simulink model "soc_WLAN_fpga"  (R2024b)
settings: Solver=FixedStepDiscrete  StartTime=0.0  StopTime=stopTime  RelTol=1e-3
PreLoadFcn:
  | addpath(fullfile(matlabroot,'toolbox','whdl','whdlexamples','whdlexamples'));
InitFcn:
  | addpath(fullfile(matlabroot,'toolbox','whdl','whdlexamples','whdlexamples'));
model workspace (MAT data in the model file):
  socvcb : containers.Map (value not decoded)
undefined symbols (not defined in the file): Add, bitRatePerOfdmSym, chanBW, coe, cpLen, dataUpsampleFactor, DelayValMaxNsdMinusLastPilotSc, DescramblerInitialSeed, designMultirateFIR, fftLen, filterLatency, filterUpsampleFactor, Fs, Hd, HT_MFMCS0, HT_MFMCS1, HT_MFMCS2, HT_MFMCS3, HT_MFMCS4, HT_MFMCS5, HT_MFMCS6, HT_MFMCS7, HTUnUsedScInd, inputSamplingRate, interp_coeff, maxPilotRefCounterVale, maxPilotsRef, maxPilotsRefNonHT, Ncol_HT, Ncol_NonHT, noDataSubCarriers, Non_HTMCS0, Non_HTMCS1, Non_HTMCS2, Non_HTMCS3, Non_HTMCS4, Non_HTMCS5, Non_HTMCS6, Non_HTMCS7, Nrow_HT, Nrow_NonHT, numDSC_HT, numDSC_HT_vhtSigB, numDSC_NonHT, numDscHT, numDscNonHT, numOfBitsPerOFDMSym, numOfDataBitsPerOFDMSym, numPilots, numScHT, numSCS_HT, numSCS_NonHT, pnSeq, QAM, rxDownsampleFactor, secondPIdx_HT, secondPIdx_NonHT, Shift, VHTMCS0, VHTMCS1 ... (+7)
libraries: hdlsllib x267, simulink x210, dspsigops x22, whdlutilities x10, whdlmod x9, dsphdlfiltering2 x5, dsphdlmathfun2 x4, whdledac x3, hwlogicconnlib x2, commhdlcrc x2, dsphdlsigops2 x2
(part 7 of 14)

== system soc_WLAN_fpga/WLAN/WLAN HDL/WLAN_Tx_Rx/WLAN_Rx/WLANHDLReceiver/DataRecovery/Decoder/Depuncturer/DepuncturerCtrlGen ==
  format : Inport
  vitInputLen : Inport  Port=2
  rstIn : Inport  Port=3
  validIn : Inport  Port=4
  Add : Sum  Inputs=+-
  Compare To Constant : simulink/Logic and Bit Operations/Compare To Constant  relop===  const=2  OutDataTypeStr=boolean
  Compare To Constant1 : simulink/Logic and Bit Operations/Compare To Constant  relop===  const=numDSC_HT_vhtSigB-1  OutDataTypeStr=boolean
  Compare To Constant2 : simulink/Logic and Bit Operations/Compare To Constant  relop===  const=numDSC_HT_vhtSigB  OutDataTypeStr=boolean
  Compare To Constant4 : simulink/Logic and Bit Operations/Compare To Constant  relop=<=  const=numDSC_HT_vhtSigB-1  OutDataTypeStr=boolean
  Compare To Zero : simulink/Logic and Bit Operations/Compare To Zero  relop===  OutDataTypeStr=boolean
  Constant : Constant  Value=fi(1,0,1,0)  SampleTime=-1
  Constant1 : Constant  Value=numDSC_HT_vhtSigB  OutDataTypeStr=fixdt(0,17,0)  SampleTime=-1
  HDL Counter : hdlsllib/Sources/HDL Counter  CountType=Count limited  CountInit=0  CountStep=1  CountMax=65535  CountFromType=Initial value  CountFrom=0  CountResetPort=on  CountLoadPort=off  CountEnbPort=on  CountDirPort=off  CountHitOutputPort=off  CountDataType=Unsigned  CountWordLen=16  CountFracLen=0  CountSampTime=1
  Logical Operator{,1..2,5,7} (5 alike) : Logic  AllPortsSameDT=off  OutDataTypeStr=boolean
  Logical Operator3 : Logic  Operator=OR  AllPortsSameDT=off  OutDataTypeStr=boolean
  Logical Operator6 : Logic  Operator=OR  AllPortsSameDT=off  OutDataTypeStr=boolean
  Relational Operator : RelationalOperator  Operator===  OutDataTypeStr=boolean  RndMeth=Simplest  InputSameDT=off
  Switch2 : Switch  Criteria=u2 > Threshold  SaturateOnIntegerOverflow=off  InputSameDT=off
  start : Outport
  end : Outport  Port=2
  wires:
  Switch2/1 -> Add/1
  Logical Operator/1 -> end/1
  Logical Operator1/1 -> start/1
  vitInputLen/1 -> Switch2/3
  validIn/1 -> Logical Operator1/2, Logical Operator/2, HDL Counter/2
  rstIn/1 -> HDL Counter/1
  Logical Operator2/1 -> Logical Operator3/1
  Constant/1 -> Add/2
  HDL Counter/1 -> Compare To Zero/1, Compare To Constant4/1, Relational Operator/2, Compare To Constant2/1, Compare To Constant1/1
  Constant1/1 -> Switch2/1
  Logical Operator6/1 -> Logical Operator1/1
  Compare To Constant2/1 -> Logical Operator5/2
  Logical Operator5/1 -> Logical Operator6/1
  Relational Operator/1 -> Logical Operator3/2
  Compare To Zero/1 -> Logical Operator6/2
  Compare To Constant4/1 -> Logical Operator7/1
  format/1 -> Compare To Constant/1
  Logical Operator3/1 -> Logical Operator/1
  Logical Operator7/1 -> Switch2/2
  Compare To Constant1/1 -> Logical Operator2/2
  Add/1 -> Relational Operator/1
  Compare To Constant/1 -> Logical Operator7/2, Logical Operator5/1, Logical Operator2/1

== system soc_WLAN_fpga/WLAN/WLAN HDL/WLAN_Tx_Rx/WLAN_Rx/WLANHDLReceiver/DataRecovery/Decoder/vhtSigB/vhtSigBDecoding ==
  note: Calculating PSDU len for VHT frame using initial 25bits of VHT SigB
  note: Dectecting CRC on first 19 bits
  MCS : Inport
  rst : Inport  Port=2
  bit : Inport  Port=3
  format : Inport  Port=4
  valid : Inport  Port=5
  Compare To Constant : simulink/Logic and Bit Operations/Compare To Constant  relop===  const=2  OutDataTypeStr=boolean
  Compare To Constant1 : simulink/Logic and Bit Operations/Compare To Constant  relop=<=  const=25  OutDataTypeStr=boolean
  Compare To Constant2 : simulink/Logic and Bit Operations/Compare To Constant  relop=<=  const=19+double(chanBW==2)  OutDataTypeStr=boolean
  Compare To Constant3 : simulink/Logic and Bit Operations/Compare To Constant  relop===  const=0  OutDataTypeStr=boolean
  Compare To Constant4 : simulink/Logic and Bit Operations/Compare To Constant  relop===  const=19+double(chanBW==2)  OutDataTypeStr=boolean
  Compare To Constant5 : simulink/Logic and Bit Operations/Compare To Constant  relop=>  const=19+double(chanBW==2)  OutDataTypeStr=boolean
  Delay : Delay  DelayLength=1
  Delay1 : Delay  DelayLength=1
  Delay3 : Delay  DelayLength=1
  Delay5 : Delay  DelayLength=9
  General CRC Generator HDL Optimized : commhdlcrc/General CRC Generator HDL Optimized  Polynomial=[1 0 0 0 0 0 1 1 1]  InitialState=1  DirectMethod=on  ReflectInput=off  ReflectCRCChecksum=off  FinalXORValue=1  SimulateUsing=Code generation
  HDL Counter : hdlsllib/Sources/HDL Counter  CountType=Count limited  CountInit=0  CountStep=1  CountMax=65535  CountFromType=Initial value  CountFrom=0  CountResetPort=on  CountLoadPort=off  CountEnbPort=on  CountDirPort=off  CountHitOutputPort=off  CountDataType=Unsigned  CountWordLen=16  CountFracLen=0  CountSampTime=1
  HDL Counter1 : hdlsllib/Sources/HDL Counter  CountType=Count limited  CountInit=0  CountStep=1  CountMax=65535  CountFromType=Initial value  CountFrom=0  CountResetPort=on  CountLoadPort=off  CountEnbPort=on  CountDirPort=off  CountHitOutputPort=off  CountDataType=Unsigned  CountWordLen=16  CountFracLen=0  CountSampTime=1
  Logical Operator{,1..3} (4 alike) : Logic  Inputs=3  AllPortsSameDT=off  OutDataTypeStr=boolean
  Logical Operator4 : Logic  AllPortsSameDT=off  OutDataTypeStr=boolean
  Shift Arithmetic : ArithShift  BitShiftNumber=2  BitShiftDirection=Left
  Terminator1 : Terminator
  Terminator3 : Terminator
  To Workspace : ToWorkspace  VariableName=vhtSigBits  SampleTime=-1
      settings: Save2DSignal=2-D array (concatenate along first dimension)
  To Workspace1 : ToWorkspace  VariableName=vhtSigBitsV  SampleTime=-1
      settings: Save2DSignal=2-D array (concatenate along first dimension)
  interpretVHTSigB : MATLAB Function  TreatAsAtomicUnit=on
  vitInputLenCalc : Subsystem
  vitInputLen : Outport
  psduLen : Outport  Port=2
  vhtCRCRefBits : Outport  Port=3
  vhtCRCRefBitValid : Outport  Port=4
  vhtSigBBitVld : Outport  Port=5
  wires:
  format/1 -> Compare To Constant/1
  valid/1 -> Logical Operator3/2, Logical Operator1/2, Logical Operator2/2, Logical Operator/3, HDL Counter/2
  rst/1 -> HDL Counter1/1, interpretVHTSigB/4(reset), HDL Counter/1
  bit/1 -> General CRC Generator HDL Optimized/1, To Workspace/1, interpretVHTSigB/1(bit)
  interpretVHTSigB/1(psduLen) -> Shift Arithmetic/1
  Compare To Constant1/1 -> Logical Operator/2
  HDL Counter/1 -> Compare To Constant1/1, Compare To Constant2/1, Compare To Constant3/1, Compare To Constant4/1, interpretVHTSigB/3(countVal)
  Compare To Constant2/1 -> Logical Operator1/3
  Logical Operator1/1 -> General CRC Generator HDL Optimized/4
  Compare To Constant3/1 -> Logical Operator2/3
  Logical Operator2/1 -> General CRC Generator HDL Optimized/2
  Logical Operator3/1 -> General CRC Generator HDL Optimized/3
  Compare To Constant4/1 -> Logical Operator3/3
  Compare To Constant/1 -> Logical Operator2/1, Logical Operator1/1, Logical Operator3/1, Logical Operator/1
  General CRC Generator HDL Optimized/4 -> Logical Operator4/1, HDL Counter1/2
  vitInputLenCalc/2(decoderInpLen) -> vitInputLen/1
  vitInputLenCalc/1(updatedPsduLen) -> psduLen/1
  MCS/1 -> Delay/1
  Shift Arithmetic/1 -> Delay1/1
  Logical Operator/1 -> Delay3/1, To Workspace1/1, interpretVHTSigB/2(validIn)
  Delay/1 -> vitInputLenCalc/1(MCS)
  Delay1/1 -> vitInputLenCalc/2(psduLen)
  Delay3/1 -> Delay5/1
  Delay5/1 -> vhtSigBBitVld/1
  General CRC Generator HDL Optimized/2 -> Terminator1/1
  General CRC Generator HDL Optimized/3 -> Terminator3/1
  General CRC Generator HDL Optimized/1 -> vhtCRCRefBits/1
  HDL Counter1/1 -> Compare To Constant5/1
  Compare To Constant5/1 -> Logical Operator4/2
  Logical Operator4/1 -> vhtCRCRefBitValid/1

== system soc_WLAN_fpga/WLAN/WLAN HDL/WLAN_Tx_Rx/WLAN_Rx/WLANHDLReceiver/DataRecovery/Deinterleaver/DeInterleaver_HT/Stage 2 16QAM  ==
  note: Give null output if valid is LOW
  dataIn : Inport
  startIn : Inport  Port=2
  endIn : Inport  Port=3
  validIn : Inport  Port=4
  Constant : Constant  Value=0  OutDataTypeStr=Inherit: Inherit via back propagation  SampleTime=-1
  Delay{1,3..6,9..11} (8 alike) : Delay  DelayLength=1
  Delay12 : Delay  DelayLength=7
  Delay13 : Delay  DelayLength=7
  Delay14 : Delay  DelayLength=7
  Delay{2,15..17} (4 alike) : Delay
  Delay7 : Delay  DelayLength=1  InitialCondition=true
  Delay8 : Delay  DelayLength=1  InitialCondition=true
  Generate Ready : Subsystem
  Logical Operator : Logic  IconShape=distinctive  AllPortsSameDT=off  OutDataTypeStr=boolean
  RAM : hdlsllib/HDL RAMs/Simple Dual Port RAM  ram_size=nextpow2(2*maxBlkSize)
  Read Logic : Subsystem
  Store Block Lengths : hdlsllib/HDL RAMs/HDL FIFO  fifo_size=4  mode=Classic  ratio=1  push_msg=Warning  pop_msg=Ignore  show_empty=off  show_full=off  show_num=on  LabelModeActiveChoice_Mode=Classic  rst_port=off
  Switch : Switch  Criteria=u2 ~= 0  SaturateOnIntegerOverflow=off
  Write Logic : Subsystem
  dataOut : Outport
  startOut : Outport  Port=2
  endOut : Outport  Port=3
  validOut : Outport  Port=4
  ready : Outport  Port=5
  wires:
  Delay17/1 -> Delay14/1
  Delay16/1 -> Delay12/1
  Delay15/1 -> Delay13/1
  Delay14/1 -> RAM/1
  Delay12/1 -> RAM/2
  Delay13/1 -> RAM/3
  Constant/1 -> Switch/3
  Switch/1 -> dataOut/1
  RAM/1 -> Switch/1
  Generate Ready/1(ready) -> ready/1, [ready]
  Read Logic/6(advPop) -> Generate Ready/1(advPop)
  Write Logic/5(endReady) -> Generate Ready/4(endReady)
  Delay7/1 -> Logical Operator/2
  validIn/1 -> Logical Operator/1
  Logical Operator/1 -> Write Logic/2(valid)
  [ready] -> Delay7/1
  Read Logic/5(pop) -> [b]
  Delay6/1 -> startOut/1
  Delay10/1 -> validOut/1, Switch/2
  Delay5/1 -> endOut/1
  Delay11/1 -> Store Block Lengths/2
  Delay9/1 -> Store Block Lengths/1
  Delay4/1 -> Delay15/1
  Delay3/1 -> Delay16/1
  Delay1/1 -> Delay17/1
  Delay8/1 -> Store Block Lengths/3, Generate Ready/3(pop)
  [b] -> Delay8/1
  Read Logic/3(end) -> Delay5/1
  Read Logic/2(start) -> Delay6/1
  Read Logic/1(rdAddr) -> RAM/4
  Store Block Lengths/1 -> Read Logic/1(fifoData)
  Read Logic/4(valid) -> Delay10/1
  Write Logic/4(endOut) -> Delay11/1
  Write Logic/3(count) -> Delay9/1
  Write Logic/2(wrValid) -> Delay4/1
  Write Logic/1(wrAddr) -> Delay3/1
  endIn/1 -> Write Logic/3(end)
  startIn/1 -> Write Logic/1(start)
  Delay2/1 -> Delay1/1
  dataIn/1 -> Delay2/1
  Store Block Lengths/2 -> Read Logic/2(fifoCount), Generate Ready/2(fifoCount)

== system soc_WLAN_fpga/WLAN/WLAN HDL/WLAN_Tx_Rx/WLAN_Rx/WLANHDLReceiver/DataRecovery/Deinterleaver/DeInterleaver_HT/Stage 2 64QAM ==
  note: Give null output if valid is LOW
  dataIn : Inport
  startIn : Inport  Port=2
  endIn : Inport  Port=3
  validIn : Inport  Port=4
  Constant : Constant  Value=0  OutDataTypeStr=Inherit: Inherit via back propagation  SampleTime=-1
  Delay{1,3..6,9..11} (8 alike) : Delay  DelayLength=1
  Delay12 : Delay  DelayLength=7
  Delay13 : Delay  DelayLength=7
  Delay14 : Delay  DelayLength=7
  Delay{2,15..17} (4 alike) : Delay
  Delay7 : Delay  DelayLength=1  InitialCondition=true
  Delay8 : Delay  DelayLength=1  InitialCondition=true
  Generate Ready : Subsystem
  Logical Operator : Logic  IconShape=distinctive  AllPortsSameDT=off  OutDataTypeStr=boolean
  RAM : hdlsllib/HDL RAMs/Simple Dual Port RAM  ram_size=nextpow2(2*maxBlkSize)
  Read Logic : Subsystem
  Store Block Lengths : hdlsllib/HDL RAMs/HDL FIFO  fifo_size=4  mode=Classic  ratio=1  push_msg=Warning  pop_msg=Ignore  show_empty=off  show_full=off  show_num=on  LabelModeActiveChoice_Mode=Classic  rst_port=off
  Switch : Switch  Criteria=u2 ~= 0  SaturateOnIntegerOverflow=off
  Write Logic : Subsystem
  dataOut : Outport
  startOut : Outport  Port=2
  endOut : Outport  Port=3
  validOut : Outport  Port=4
  ready : Outport  Port=5
  wires:
  Delay17/1 -> Delay14/1
  Delay16/1 -> Delay12/1
  Delay15/1 -> Delay13/1
  Delay14/1 -> RAM/1
  Delay12/1 -> RAM/2
  Delay13/1 -> RAM/3
  Constant/1 -> Switch/3
  Switch/1 -> dataOut/1
  RAM/1 -> Switch/1
  Generate Ready/1(ready) -> ready/1, [ready]
  Read Logic/6(advPop) -> Generate Ready/1(advPop)
  Write Logic/5(endReady) -> Generate Ready/4(endReady)
  Delay7/1 -> Logical Operator/2
  validIn/1 -> Logical Operator/1
  Logical Operator/1 -> Write Logic/2(valid)
  [ready] -> Delay7/1
  Read Logic/5(pop) -> [b]
  Delay6/1 -> startOut/1
  Delay10/1 -> validOut/1, Switch/2
  Delay5/1 -> endOut/1
  Delay11/1 -> Store Block Lengths/2
  Delay9/1 -> Store Block Lengths/1
  Delay4/1 -> Delay15/1
  Delay3/1 -> Delay16/1
  Delay1/1 -> Delay17/1
  Delay8/1 -> Store Block Lengths/3, Generate Ready/3(pop)
  [b] -> Delay8/1
  Read Logic/3(end) -> Delay5/1
  Read Logic/2(start) -> Delay6/1
  Read Logic/1(rdAddr) -> RAM/4
  Store Block Lengths/1 -> Read Logic/1(fifoData)
  Read Logic/4(valid) -> Delay10/1
  Write Logic/4(endOut) -> Delay11/1
  Write Logic/3(count) -> Delay9/1
  Write Logic/2(wrValid) -> Delay4/1
  Write Logic/1(wrAddr) -> Delay3/1
  endIn/1 -> Write Logic/3(end)
  startIn/1 -> Write Logic/1(start)
  Delay2/1 -> Delay1/1
  dataIn/1 -> Delay2/1
  Store Block Lengths/2 -> Read Logic/2(fifoCount), Generate Ready/2(fifoCount)

== system soc_WLAN_fpga/WLAN/WLAN HDL/WLAN_Tx_Rx/WLAN_Rx/WLANHDLReceiver/DataRecovery/Deinterleaver/DeInterleaver_HT/Stage 2 BPSK ==
  note: Give null output if valid is LOW
  dataIn : Inport
  startIn : Inport  Port=2
  endIn : Inport  Port=3
  validIn : Inport  Port=4
  Constant : Constant  Value=0  OutDataTypeStr=Inherit: Inherit via back propagation  SampleTime=-1
  Delay{1,3..6,9..11} (8 alike) : Delay  DelayLength=1
  Delay12 : Delay  DelayLength=7
  Delay13 : Delay  DelayLength=7
  Delay14 : Delay  DelayLength=7
  Delay{2,15..17} (4 alike) : Delay
  Delay7 : Delay  DelayLength=1  InitialCondition=true
  Delay8 : Delay  DelayLength=1  InitialCondition=true
  Generate Ready : Subsystem
  Logical Operator : Logic  IconShape=distinctive  AllPortsSameDT=off  OutDataTypeStr=boolean
  RAM : hdlsllib/HDL RAMs/Simple Dual Port RAM  ram_size=nextpow2(2*maxBlkSize)
  Read Logic : Subsystem
  Store Block Lengths : hdlsllib/HDL RAMs/HDL FIFO  fifo_size=4  mode=Classic  ratio=1  push_msg=Warning  pop_msg=Ignore  show_empty=off  show_full=off  show_num=on  LabelModeActiveChoice_Mode=Classic  rst_port=off
  Switch : Switch  Criteria=u2 ~= 0  SaturateOnIntegerOverflow=off
  Write Logic : Subsystem
  dataOut : Outport
  startOut : Outport  Port=2
  endOut : Outport  Port=3
  validOut : Outport  Port=4
  ready : Outport  Port=5
  wires:
  Delay17/1 -> Delay14/1
  Delay16/1 -> Delay12/1
  Delay15/1 -> Delay13/1
  Delay14/1 -> RAM/1
  Delay12/1 -> RAM/2
  Delay13/1 -> RAM/3
  Constant/1 -> Switch/3
  Switch/1 -> dataOut/1
  RAM/1 -> Switch/1
  Generate Ready/1(ready) -> ready/1, [ready]
  Read Logic/6(advPop) -> Generate Ready/1(advPop)
  Write Logic/5(endReady) -> Generate Ready/4(endReady)
  Delay7/1 -> Logical Operator/2
  validIn/1 -> Logical Operator/1
  Logical Operator/1 -> Write Logic/2(valid)
  [ready] -> Delay7/1
  Read Logic/5(pop) -> [b]
  Delay6/1 -> startOut/1
  Delay10/1 -> validOut/1, Switch/2
  Delay5/1 -> endOut/1
  Delay11/1 -> Store Block Lengths/2
  Delay9/1 -> Store Block Lengths/1
  Delay4/1 -> Delay15/1
  Delay3/1 -> Delay16/1
  Delay1/1 -> Delay17/1
  Delay8/1 -> Store Block Lengths/3, Generate Ready/3(pop)
  [b] -> Delay8/1
  Read Logic/3(end) -> Delay5/1
  Read Logic/2(start) -> Delay6/1
  Read Logic/1(rdAddr) -> RAM/4
  Store Block Lengths/1 -> Read Logic/1(fifoData)
  Read Logic/4(valid) -> Delay10/1
  Write Logic/4(endOut) -> Delay11/1
  Write Logic/3(count) -> Delay9/1
  Write Logic/2(wrValid) -> Delay4/1
  Write Logic/1(wrAddr) -> Delay3/1
  endIn/1 -> Write Logic/3(end)
  startIn/1 -> Write Logic/1(start)
  Delay2/1 -> Delay1/1
  dataIn/1 -> Delay2/1
  Store Block Lengths/2 -> Read Logic/2(fifoCount), Generate Ready/2(fifoCount)

== system soc_WLAN_fpga/WLAN/WLAN HDL/WLAN_Tx_Rx/WLAN_Rx/WLANHDLReceiver/DataRecovery/Deinterleaver/DeInterleaver_HT/Stage 2 QPSK ==
  note: Give null output if valid is LOW
  dataIn : Inport
  startIn : Inport  Port=2
  endIn : Inport  Port=3
  validIn : Inport  Port=4
  Constant : Constant  Value=0  OutDataTypeStr=Inherit: Inherit via back propagation  SampleTime=-1
  Delay{1,3..6,9..11} (8 alike) : Delay  DelayLength=1
  Delay12 : Delay  DelayLength=7
  Delay13 : Delay  DelayLength=7
  Delay14 : Delay  DelayLength=7
  Delay{2,15..17} (4 alike) : Delay
  Delay7 : Delay  DelayLength=1  InitialCondition=true
  Delay8 : Delay  DelayLength=1  InitialCondition=true
  Generate Ready : Subsystem
  Logical Operator : Logic  IconShape=distinctive  AllPortsSameDT=off  OutDataTypeStr=boolean
  RAM : hdlsllib/HDL RAMs/Simple Dual Port RAM  ram_size=nextpow2(2*maxBlkSize)
  Read Logic : Subsystem
  Store Block Lengths : hdlsllib/HDL RAMs/HDL FIFO  fifo_size=4  mode=Classic  ratio=1  push_msg=Warning  pop_msg=Ignore  show_empty=off  show_full=off  show_num=on  LabelModeActiveChoice_Mode=Classic  rst_port=off
  Switch : Switch  Criteria=u2 ~= 0  SaturateOnIntegerOverflow=off
  Write Logic : Subsystem
  dataOut : Outport
  startOut : Outport  Port=2
  endOut : Outport  Port=3
  validOut : Outport  Port=4
  ready : Outport  Port=5
  wires:
  Delay17/1 -> Delay14/1
  Delay16/1 -> Delay12/1
  Delay15/1 -> Delay13/1
  Delay14/1 -> RAM/1
  Delay12/1 -> RAM/2
  Delay13/1 -> RAM/3
  Constant/1 -> Switch/3
  Switch/1 -> dataOut/1
  RAM/1 -> Switch/1
  Generate Ready/1(ready) -> ready/1, [ready]
  Read Logic/6(advPop) -> Generate Ready/1(advPop)
  Write Logic/5(endReady) -> Generate Ready/4(endReady)
  Delay7/1 -> Logical Operator/2
  validIn/1 -> Logical Operator/1
  Logical Operator/1 -> Write Logic/2(valid)
  [ready] -> Delay7/1
  Read Logic/5(pop) -> [b]
  Delay6/1 -> startOut/1
  Delay10/1 -> validOut/1, Switch/2
  Delay5/1 -> endOut/1
  Delay11/1 -> Store Block Lengths/2
  Delay9/1 -> Store Block Lengths/1
  Delay4/1 -> Delay15/1
  Delay3/1 -> Delay16/1
  Delay1/1 -> Delay17/1
  Delay8/1 -> Store Block Lengths/3, Generate Ready/3(pop)
  [b] -> Delay8/1
  Read Logic/3(end) -> Delay5/1
  Read Logic/2(start) -> Delay6/1
  Read Logic/1(rdAddr) -> RAM/4
  Store Block Lengths/1 -> Read Logic/1(fifoData)
  Read Logic/4(valid) -> Delay10/1
  Write Logic/4(endOut) -> Delay11/1
  Write Logic/3(count) -> Delay9/1
  Write Logic/2(wrValid) -> Delay4/1
  Write Logic/1(wrAddr) -> Delay3/1
  endIn/1 -> Write Logic/3(end)
  startIn/1 -> Write Logic/1(start)
  Delay2/1 -> Delay1/1
  dataIn/1 -> Delay2/1
  Store Block Lengths/2 -> Read Logic/2(fifoCount), Generate Ready/2(fifoCount)

== system soc_WLAN_fpga/WLAN/WLAN HDL/WLAN_Tx_Rx/WLAN_Rx/WLANHDLReceiver/DataRecovery/Deinterleaver/DeInterleaver_HT/Stage1 ==
  wr_din : Inport
  enb : Inport  Port=2
  bps : Inport  Port=3
  rst : Inport  Port=4
  numSCs : Inport  Port=5
  2-D Lookup Table : Lookup_n-D  BreakpointsForDimension1=1:4  BreakpointsForDimension2=0:length(secondPIdx_HT)-1  IndexSearchMethod=Evenly spaced points  Table=uint16(secondPIdx_HT-1)  ExtrapMethod=Clip  UseLastTableValue=on  InternalRulePriority=Speed  OutDataTypeStr=uint16  RndMeth=Simplest
      settings: InputPortMap=u0,u1
  Compare To Constant1 : simulink/Logic and Bit Operations/Compare To Constant  relop===  const=0  OutDataTypeStr=boolean
  Compare To Zero : simulink/Logic and Bit Operations/Compare To Zero  relop=>  OutDataTypeStr=boolean
  Constant : Constant  OutDataTypeStr=uint16  SampleTime=-1
  Delay : Delay  DelayLength=52
  Delay1 : Delay  DelayLength=1  InputProcessing=Columns as channels (frame based)
  Delay{2..9} (8 alike) : Delay  DelayLength=1
  HDL Counter : hdlsllib/Sources/HDL Counter  CountType=Count limited  CountInit=0  CountStep=1  CountMax=length(secondPIdx_HT)-1  CountFromType=Initial value  CountFrom=0  CountResetPort=on  CountLoadPort=off  CountEnbPort=on  CountDirPort=off  CountHitOutputPort=off  CountDataType=Unsigned  CountWordLen=16  CountFracLen=0  CountSampTime=1
  HDL Counter1 : hdlsllib/Sources/HDL Counter  CountType=Count limited  CountInit=0  CountStep=1  CountMax=1  CountFromType=Initial value  CountFrom=0  CountResetPort=on  CountLoadPort=off  CountEnbPort=on  CountDirPort=off  CountHitOutputPort=off  CountDataType=Unsigned  CountWordLen=1  CountFracLen=0  CountSampTime=1
  HDL Counter2 : hdlsllib/Sources/HDL Counter  CountType=Count limited  CountInit=0  CountStep=1  CountMax=length(secondPIdx_HT)-1  CountFromType=Initial value  CountFrom=0  CountResetPort=on  CountLoadPort=on  CountEnbPort=on  CountDirPort=off  CountHitOutputPort=off  CountDataType=Unsigned  CountWordLen=16  CountFracLen=0  CountSampTime=1
  Logical Operator : Logic  AllPortsSameDT=off  OutDataTypeStr=boolean
  Logical Operator1 : Logic  AllPortsSameDT=off  OutDataTypeStr=boolean
  Logical Operator2 : Logic  Operator=NOT  AllPortsSameDT=off  OutDataTypeStr=boolean
  Logical Operator3 : Logic  Operator=OR  AllPortsSameDT=off  OutDataTypeStr=boolean
  Logical Operator4 : Logic  Operator=OR  AllPortsSameDT=off  OutDataTypeStr=boolean
  Logical Operator5 : Logic  Operator=OR  AllPortsSameDT=off  OutDataTypeStr=boolean
  Logical Operator6 : Logic  AllPortsSameDT=off  OutDataTypeStr=boolean
  Relational Operator : RelationalOperator  Operator===  OutDataTypeStr=boolean  RndMeth=Simplest  InputSameDT=off
  Relational Operator1 : RelationalOperator  Operator===  OutDataTypeStr=boolean  RndMeth=Simplest  InputSameDT=off
  Simple Dual Port RAM : hdlsllib/HDL RAMs/Simple Dual Port RAM  ram_size=16
  Simple Dual Port RAM1 : hdlsllib/HDL RAMs/Simple Dual Port RAM  ram_size=16
  Switch : Switch  Criteria=u2 > Threshold  SaturateOnIntegerOverflow=off  InputSameDT=off
  dataOut : Outport
  validOut : Outport  Port=2
  wires:
  enb/1 -> HDL Counter/2, Logical Operator6/1, Logical Operator/1, Logical Operator1/1
  Simple Dual Port RAM/1 -> Switch/1
  bps/1 -> 2-D Lookup Table/1
  HDL Counter/1 -> Delay3/1, Relational Operator/1, Delay6/1
  HDL Counter1/1 -> Compare To Constant1/1
  wr_din/1 -> Delay2/1
  Relational Operator/1 -> Logical Operator6/2
  Logical Operator1/1 -> Delay7/1
  2-D Lookup Table/1 -> Delay8/1
  rst/1 -> HDL Counter1/1, Logical Operator4/1, Logical Operator3/1
  Simple Dual Port RAM1/1 -> Switch/3
  Logical Operator/1 -> Delay4/1
  Switch/1 -> dataOut/1
  Delay1/1 -> validOut/1
  HDL Counter2/1 -> Compare To Zero/1, Relational Operator1/1, 2-D Lookup Table/2
  Compare To Constant1/1 -> Logical Operator/2, Logical Operator2/1
  numSCs/1 -> Delay/1, Relational Operator/2
  Relational Operator1/1 -> Logical Operator3/2
  Logical Operator3/1 -> HDL Counter2/1
  Logical Operator4/1 -> HDL Counter/1
  Constant/1 -> HDL Counter2/3
  Compare To Zero/1 -> Logical Operator5/2, HDL Counter2/4
  Logical Operator5/1 -> Delay9/1
  Logical Operator2/1 -> Logical Operator1/2, Delay5/1
  Logical Operator6/1 -> HDL Counter1/2, Logical Operator5/1, HDL Counter2/2, Logical Operator4/2
  Delay2/1 -> Simple Dual Port RAM1/1, Simple Dual Port RAM/1
  Delay3/1 -> Simple Dual Port RAM/2
  Delay4/1 -> Simple Dual Port RAM/3
  Delay5/1 -> Switch/2
  Delay6/1 -> Simple Dual Port RAM1/2
  Delay7/1 -> Simple Dual Port RAM1/3
  Delay8/1 -> Simple Dual Port RAM/4, Simple Dual Port RAM1/4
  Delay9/1 -> Delay1/1
  Delay/1 -> Relational Operator1/2

== system soc_WLAN_fpga/WLAN/WLAN HDL/WLAN_Tx_Rx/WLAN_Rx/WLANHDLReceiver/DataRecovery/Deinterleaver/DeInterleaver_HT/ctrlGen ==
  enb : Inport
  numSCsIn : Inport  Port=2
  rst : Inport  Port=3
  Compare To Zero : simulink/Logic and Bit Operations/Compare To Zero  relop===  OutDataTypeStr=boolean
  HDL Counter : hdlsllib/Sources/HDL Counter  CountType=Count limited  CountInit=0  CountStep=1  CountMax=length(secondPIdx_HT)-1  CountFromType=Initial value  CountFrom=0  CountResetPort=on  CountLoadPort=off  CountEnbPort=on  CountDirPort=off  CountHitOutputPort=off  CountDataType=Unsigned  CountWordLen=16  CountFracLen=0  CountSampTime=1
  Logical Operator : Logic  AllPortsSameDT=off  OutDataTypeStr=boolean
  Logical Operator1 : Logic  AllPortsSameDT=off  OutDataTypeStr=boolean
  Logical Operator2 : Logic  Operator=OR  AllPortsSameDT=off  OutDataTypeStr=boolean
  Relational Operator : RelationalOperator  Operator===  OutDataTypeStr=boolean  RndMeth=Simplest  InputSameDT=off
  Out1 : Outport
  Out2 : Outport  Port=2
  wires:
  Logical Operator/1 -> Out2/1
  HDL Counter/1 -> Relational Operator/1, Compare To Zero/1
  Logical Operator1/1 -> Out1/1
  Compare To Zero/1 -> Logical Operator1/2
  enb/1 -> Logical Operator1/1, HDL Counter/2, Logical Operator/2
  Relational Operator/1 -> Logical Operator2/2, Logical Operator/1
  numSCsIn/1 -> Relational Operator/2
  Logical Operator2/1 -> HDL Counter/1
  rst/1 -> Logical Operator2/1

== system soc_WLAN_fpga/WLAN/WLAN HDL/WLAN_Tx_Rx/WLAN_Rx/WLANHDLReceiver/DataRecovery/Deinterleaver/DeInterleaver_HT/numSCsConverter ==
  numSCS : Inport
  bps : Inport  Port=2
  Add : Sum  Inputs=+-
  Add1 : Sum  Inputs=+-
  Add2 : Sum  Inputs=+-
  Add3 : Sum  OutDataTypeStr=fixdt(0,9,0)
  Constant1 : Constant  Value=fi(1,0,1,0)  SampleTime=-1
  Constant3 : Constant  Value=fi(6,0,3,0)  SampleTime=-1
  Multiport Switch5 : MultiPortSwitch  Inputs=4  SaturateOnIntegerOverflow=off  InputSameDT=off
  Product : Product
  Shift Arithmetic : ArithShift  BitShiftNumber=1  BitShiftDirection=Left
  Shift Arithmetic1 : ArithShift  BitShiftNumber=2  BitShiftDirection=Left
  numSCSOut : Outport
  wires:
  Shift Arithmetic/1 -> Add/1
  Multiport Switch5/1 -> numSCSOut/1
  Add2/1 -> Multiport Switch5/5
  Constant1/1 -> Add/2, Add2/2, Add3/2, Add1/2
  bps/1 -> Multiport Switch5/1
  Add1/1 -> Multiport Switch5/4
  Add/1 -> Multiport Switch5/3
  Shift Arithmetic1/1 -> Add1/1
  Constant3/1 -> Product/2
  Product/1 -> Add2/1
  Add3/1 -> Product/1, Shift Arithmetic1/1, Shift Arithmetic/1
  numSCS/1 -> Multiport Switch5/2, Add3/1

== system soc_WLAN_fpga/WLAN/WLAN HDL/WLAN_Tx_Rx/WLAN_Rx/WLANHDLReceiver/DataRecovery/Deinterleaver/DeInterleaver_NonHT/Stage 2 16QAM  ==
  note: Give null output if valid is LOW
  dataIn : Inport
  startIn : Inport  Port=2
  endIn : Inport  Port=3
  validIn : Inport  Port=4
  Constant : Constant  Value=0  OutDataTypeStr=Inherit: Inherit via back propagation  SampleTime=-1
  Delay{1,3..6,9..11} (8 alike) : Delay  DelayLength=1
  Delay12 : Delay  DelayLength=7
  Delay13 : Delay  DelayLength=7
  Delay14 : Delay  DelayLength=7
  Delay{2,15..17} (4 alike) : Delay
  Delay7 : Delay  DelayLength=1  InitialCondition=true
  Delay8 : Delay  DelayLength=1  InitialCondition=true
  Generate Ready : Subsystem
  Logical Operator : Logic  IconShape=distinctive  AllPortsSameDT=off  OutDataTypeStr=boolean
  RAM : hdlsllib/HDL RAMs/Simple Dual Port RAM  ram_size=nextpow2(2*maxBlkSize)
  Read Logic : Subsystem
  Store Block Lengths : hdlsllib/HDL RAMs/HDL FIFO  fifo_size=4  mode=Classic  ratio=1  push_msg=Warning  pop_msg=Ignore  show_empty=off  show_full=off  show_num=on  LabelModeActiveChoice_Mode=Classic  rst_port=off
  Switch : Switch  Criteria=u2 ~= 0  SaturateOnIntegerOverflow=off
  Write Logic : Subsystem
  dataOut : Outport
  startOut : Outport  Port=2
  endOut : Outport  Port=3
  validOut : Outport  Port=4
  ready : Outport  Port=5
  wires:
  Delay17/1 -> Delay14/1
  Delay16/1 -> Delay12/1
  Delay15/1 -> Delay13/1
  Delay14/1 -> RAM/1
  Delay12/1 -> RAM/2
  Delay13/1 -> RAM/3
  Constant/1 -> Switch/3
  Switch/1 -> dataOut/1
  RAM/1 -> Switch/1
  Generate Ready/1(ready) -> ready/1, [ready]
  Read Logic/6(advPop) -> Generate Ready/1(advPop)
  Write Logic/5(endReady) -> Generate Ready/4(endReady)
  Delay7/1 -> Logical Operator/2
  validIn/1 -> Logical Operator/1
  Logical Operator/1 -> Write Logic/2(valid)
  [ready] -> Delay7/1
  Read Logic/5(pop) -> [b]
  Delay6/1 -> startOut/1
  Delay10/1 -> validOut/1, Switch/2
  Delay5/1 -> endOut/1
  Delay11/1 -> Store Block Lengths/2
  Delay9/1 -> Store Block Lengths/1
  Delay4/1 -> Delay15/1
  Delay3/1 -> Delay16/1
  Delay1/1 -> Delay17/1
  Delay8/1 -> Store Block Lengths/3, Generate Ready/3(pop)
  [b] -> Delay8/1
  Read Logic/3(end) -> Delay5/1
  Read Logic/2(start) -> Delay6/1
  Read Logic/1(rdAddr) -> RAM/4
  Store Block Lengths/1 -> Read Logic/1(fifoData)
  Read Logic/4(valid) -> Delay10/1
  Write Logic/4(endOut) -> Delay11/1
  Write Logic/3(count) -> Delay9/1
  Write Logic/2(wrValid) -> Delay4/1
  Write Logic/1(wrAddr) -> Delay3/1
  endIn/1 -> Write Logic/3(end)
  startIn/1 -> Write Logic/1(start)
  Delay2/1 -> Delay1/1
  dataIn/1 -> Delay2/1
  Store Block Lengths/2 -> Read Logic/2(fifoCount), Generate Ready/2(fifoCount)

== system soc_WLAN_fpga/WLAN/WLAN HDL/WLAN_Tx_Rx/WLAN_Rx/WLANHDLReceiver/DataRecovery/Deinterleaver/DeInterleaver_NonHT/Stage 2 64QAM ==
  note: Give null output if valid is LOW
  dataIn : Inport
  startIn : Inport  Port=2
  endIn : Inport  Port=3
  validIn : Inport  Port=4
  Constant : Constant  Value=0  OutDataTypeStr=Inherit: Inherit via back propagation  SampleTime=-1
  Delay{1,3..6,9..11} (8 alike) : Delay  DelayLength=1
  Delay12 : Delay  DelayLength=7
  Delay13 : Delay  DelayLength=7
  Delay14 : Delay  DelayLength=7
  Delay{2,15..17} (4 alike) : Delay
  Delay7 : Delay  DelayLength=1  InitialCondition=true
  Delay8 : Delay  DelayLength=1  InitialCondition=true
  Generate Ready : Subsystem
  Logical Operator : Logic  IconShape=distinctive  AllPortsSameDT=off  OutDataTypeStr=boolean
  RAM : hdlsllib/HDL RAMs/Simple Dual Port RAM  ram_size=nextpow2(2*maxBlkSize)
  Read Logic : Subsystem
  Store Block Lengths : hdlsllib/HDL RAMs/HDL FIFO  fifo_size=4  mode=Classic  ratio=1  push_msg=Warning  pop_msg=Ignore  show_empty=off  show_full=off  show_num=on  LabelModeActiveChoice_Mode=Classic  rst_port=off
  Switch : Switch  Criteria=u2 ~= 0  SaturateOnIntegerOverflow=off
  Write Logic : Subsystem
  dataOut : Outport
  startOut : Outport  Port=2
  endOut : Outport  Port=3
  validOut : Outport  Port=4
  ready : Outport  Port=5
  wires:
  Delay17/1 -> Delay14/1
  Delay16/1 -> Delay12/1
  Delay15/1 -> Delay13/1
  Delay14/1 -> RAM/1
  Delay12/1 -> RAM/2
  Delay13/1 -> RAM/3
  Constant/1 -> Switch/3
  Switch/1 -> dataOut/1
  RAM/1 -> Switch/1
  Generate Ready/1(ready) -> ready/1, [ready]
  Read Logic/6(advPop) -> Generate Ready/1(advPop)
  Write Logic/5(endReady) -> Generate Ready/4(endReady)
  Delay7/1 -> Logical Operator/2
  validIn/1 -> Logical Operator/1
  Logical Operator/1 -> Write Logic/2(valid)
  [ready] -> Delay7/1
  Read Logic/5(pop) -> [b]
  Delay6/1 -> startOut/1
  Delay10/1 -> validOut/1, Switch/2
  Delay5/1 -> endOut/1
  Delay11/1 -> Store Block Lengths/2
  Delay9/1 -> Store Block Lengths/1
  Delay4/1 -> Delay15/1
  Delay3/1 -> Delay16/1
  Delay1/1 -> Delay17/1
  Delay8/1 -> Store Block Lengths/3, Generate Ready/3(pop)
  [b] -> Delay8/1
  Read Logic/3(end) -> Delay5/1
  Read Logic/2(start) -> Delay6/1
  Read Logic/1(rdAddr) -> RAM/4
  Store Block Lengths/1 -> Read Logic/1(fifoData)
  Read Logic/4(valid) -> Delay10/1
  Write Logic/4(endOut) -> Delay11/1
  Write Logic/3(count) -> Delay9/1
  Write Logic/2(wrValid) -> Delay4/1
  Write Logic/1(wrAddr) -> Delay3/1
  endIn/1 -> Write Logic/3(end)
  startIn/1 -> Write Logic/1(start)
  Delay2/1 -> Delay1/1
  dataIn/1 -> Delay2/1
  Store Block Lengths/2 -> Read Logic/2(fifoCount), Generate Ready/2(fifoCount)

== system soc_WLAN_fpga/WLAN/WLAN HDL/WLAN_Tx_Rx/WLAN_Rx/WLANHDLReceiver/DataRecovery/Deinterleaver/DeInterleaver_NonHT/Stage 2 BPSK ==
  note: Give null output if valid is LOW
  dataIn : Inport
  startIn : Inport  Port=2
  endIn : Inport  Port=3
  validIn : Inport  Port=4
  Constant : Constant  Value=0  OutDataTypeStr=Inherit: Inherit via back propagation  SampleTime=-1
  Delay{1,3..6,9..11} (8 alike) : Delay  DelayLength=1
  Delay12 : Delay  DelayLength=7
  Delay13 : Delay  DelayLength=7
  Delay14 : Delay  DelayLength=7
  Delay{2,15..17} (4 alike) : Delay
  Delay7 : Delay  DelayLength=1  InitialCondition=true
  Delay8 : Delay  DelayLength=1  InitialCondition=true
  Generate Ready : Subsystem
  Logical Operator : Logic  IconShape=distinctive  AllPortsSameDT=off  OutDataTypeStr=boolean
  RAM : hdlsllib/HDL RAMs/Simple Dual Port RAM  ram_size=nextpow2(2*maxBlkSize)
  Read Logic : Subsystem
  Store Block Lengths : hdlsllib/HDL RAMs/HDL FIFO  fifo_size=4  mode=Classic  ratio=1  push_msg=Warning  pop_msg=Ignore  show_empty=off  show_full=off  show_num=on  LabelModeActiveChoice_Mode=Classic  rst_port=off
  Switch : Switch  Criteria=u2 ~= 0  SaturateOnIntegerOverflow=off
  Write Logic : Subsystem
  dataOut : Outport
  startOut : Outport  Port=2
  endOut : Outport  Port=3
  validOut : Outport  Port=4
  ready : Outport  Port=5
  wires:
  Delay17/1 -> Delay14/1
  Delay16/1 -> Delay12/1
  Delay15/1 -> Delay13/1
  Delay14/1 -> RAM/1
  Delay12/1 -> RAM/2
  Delay13/1 -> RAM/3
  Constant/1 -> Switch/3
  Switch/1 -> dataOut/1
  RAM/1 -> Switch/1
  Generate Ready/1(ready) -> ready/1, [ready]
  Read Logic/6(advPop) -> Generate Ready/1(advPop)
  Write Logic/5(endReady) -> Generate Ready/4(endReady)
  Delay7/1 -> Logical Operator/2
  validIn/1 -> Logical Operator/1
  Logical Operator/1 -> Write Logic/2(valid)
  [ready] -> Delay7/1
  Read Logic/5(pop) -> [b]
  Delay6/1 -> startOut/1
  Delay10/1 -> validOut/1, Switch/2
  Delay5/1 -> endOut/1
  Delay11/1 -> Store Block Lengths/2
  Delay9/1 -> Store Block Lengths/1
  Delay4/1 -> Delay15/1
  Delay3/1 -> Delay16/1
  Delay1/1 -> Delay17/1
  Delay8/1 -> Store Block Lengths/3, Generate Ready/3(pop)
  [b] -> Delay8/1
  Read Logic/3(end) -> Delay5/1
  Read Logic/2(start) -> Delay6/1
  Read Logic/1(rdAddr) -> RAM/4
  Store Block Lengths/1 -> Read Logic/1(fifoData)
  Read Logic/4(valid) -> Delay10/1
  Write Logic/4(endOut) -> Delay11/1
  Write Logic/3(count) -> Delay9/1
  Write Logic/2(wrValid) -> Delay4/1
  Write Logic/1(wrAddr) -> Delay3/1
  endIn/1 -> Write Logic/3(end)
  startIn/1 -> Write Logic/1(start)
  Delay2/1 -> Delay1/1
  dataIn/1 -> Delay2/1
  Store Block Lengths/2 -> Read Logic/2(fifoCount), Generate Ready/2(fifoCount)

== system soc_WLAN_fpga/WLAN/WLAN HDL/WLAN_Tx_Rx/WLAN_Rx/WLANHDLReceiver/DataRecovery/Deinterleaver/DeInterleaver_NonHT/Stage 2 QPSK ==
  note: Give null output if valid is LOW
  dataIn : Inport
  startIn : Inport  Port=2
  endIn : Inport  Port=3
  validIn : Inport  Port=4
  Constant : Constant  Value=0  OutDataTypeStr=Inherit: Inherit via back propagation  SampleTime=-1
  Delay{1,3..6,9..11} (8 alike) : Delay  DelayLength=1
  Delay12 : Delay  DelayLength=7
  Delay13 : Delay  DelayLength=7
  Delay14 : Delay  DelayLength=7
  Delay{2,15..17} (4 alike) : Delay
  Delay7 : Delay  DelayLength=1  InitialCondition=true
  Delay8 : Delay  DelayLength=1  InitialCondition=true
  Generate Ready : Subsystem
  Logical Operator : Logic  IconShape=distinctive  AllPortsSameDT=off  OutDataTypeStr=boolean
  RAM : hdlsllib/HDL RAMs/Simple Dual Port RAM  ram_size=nextpow2(2*maxBlkSize)
  Read Logic : Subsystem
  Store Block Lengths : hdlsllib/HDL RAMs/HDL FIFO  fifo_size=4  mode=Classic  ratio=1  push_msg=Warning  pop_msg=Ignore  show_empty=off  show_full=off  show_num=on  LabelModeActiveChoice_Mode=Classic  rst_port=off
  Switch : Switch  Criteria=u2 ~= 0  SaturateOnIntegerOverflow=off
  Write Logic : Subsystem
  dataOut : Outport
  startOut : Outport  Port=2
  endOut : Outport  Port=3
  validOut : Outport  Port=4
  ready : Outport  Port=5
  wires:
  Delay17/1 -> Delay14/1
  Delay16/1 -> Delay12/1
  Delay15/1 -> Delay13/1
  Delay14/1 -> RAM/1
  Delay12/1 -> RAM/2
  Delay13/1 -> RAM/3
  Constant/1 -> Switch/3
  Switch/1 -> dataOut/1
  RAM/1 -> Switch/1
  Generate Ready/1(ready) -> ready/1, [ready]
  Read Logic/6(advPop) -> Generate Ready/1(advPop)
  Write Logic/5(endReady) -> Generate Ready/4(endReady)
  Delay7/1 -> Logical Operator/2
  validIn/1 -> Logical Operator/1
  Logical Operator/1 -> Write Logic/2(valid)
  [ready] -> Delay7/1
  Read Logic/5(pop) -> [b]
  Delay6/1 -> startOut/1
  Delay10/1 -> validOut/1, Switch/2
  Delay5/1 -> endOut/1
  Delay11/1 -> Store Block Lengths/2
  Delay9/1 -> Store Block Lengths/1
  Delay4/1 -> Delay15/1
  Delay3/1 -> Delay16/1
  Delay1/1 -> Delay17/1
  Delay8/1 -> Store Block Lengths/3, Generate Ready/3(pop)
  [b] -> Delay8/1
  Read Logic/3(end) -> Delay5/1
  Read Logic/2(start) -> Delay6/1
  Read Logic/1(rdAddr) -> RAM/4
  Store Block Lengths/1 -> Read Logic/1(fifoData)
  Read Logic/4(valid) -> Delay10/1
  Write Logic/4(endOut) -> Delay11/1
  Write Logic/3(count) -> Delay9/1
  Write Logic/2(wrValid) -> Delay4/1
  Write Logic/1(wrAddr) -> Delay3/1
  endIn/1 -> Write Logic/3(end)
  startIn/1 -> Write Logic/1(start)
  Delay2/1 -> Delay1/1
  dataIn/1 -> Delay2/1
  Store Block Lengths/2 -> Read Logic/2(fifoCount), Generate Ready/2(fifoCount)

== system soc_WLAN_fpga/WLAN/WLAN HDL/WLAN_Tx_Rx/WLAN_Rx/WLANHDLReceiver/DataRecovery/Deinterleaver/DeInterleaver_NonHT/Stage1 ==
  wr_din : Inport
  enb : Inport  Port=2
  bps : Inport  Port=3
  rst : Inport  Port=4
  numSCs : Inport  Port=5
  2-D Lookup Table : Lookup_n-D  BreakpointsForDimension1=1:4  BreakpointsForDimension2=0:length(secondPIdx_NonHT)-1  IndexSearchMethod=Evenly spaced points  Table=uint16(secondPIdx_NonHT-1)  ExtrapMethod=Clip  UseLastTableValue=on  InternalRulePriority=Speed  OutDataTypeStr=uint16  RndMeth=Simplest
      settings: InputPortMap=u0,u1
  Compare To Constant1 : simulink/Logic and Bit Operations/Compare To Constant  relop===  const=0  OutDataTypeStr=boolean
  Compare To Zero : simulink/Logic and Bit Operations/Compare To Zero  relop=>  OutDataTypeStr=boolean
  Constant : Constant  OutDataTypeStr=uint16  SampleTime=-1
  Delay : Delay  DelayLength=80+75
  Delay1 : Delay  DelayLength=1  InputProcessing=Columns as channels (frame based)
  Delay{2..9} (8 alike) : Delay  DelayLength=1
  HDL Counter : hdlsllib/Sources/HDL Counter  CountType=Count limited  CountInit=0  CountStep=1  CountMax=length(secondPIdx_NonHT)-1  CountFromType=Initial value  CountFrom=0  CountResetPort=on  CountLoadPort=off  CountEnbPort=on  CountDirPort=off  CountHitOutputPort=off  CountDataType=Unsigned  CountWordLen=16  CountFracLen=0  CountSampTime=1
  HDL Counter1 : hdlsllib/Sources/HDL Counter  CountType=Count limited  CountInit=0  CountStep=1  CountMax=1  CountFromType=Initial value  CountFrom=0  CountResetPort=on  CountLoadPort=off  CountEnbPort=on  CountDirPort=off  CountHitOutputPort=off  CountDataType=Unsigned  CountWordLen=1  CountFracLen=0  CountSampTime=1
  HDL Counter2 : hdlsllib/Sources/HDL Counter  CountType=Count limited  CountInit=0  CountStep=1  CountMax=length(secondPIdx_NonHT)-1  CountFromType=Initial value  CountFrom=0  CountResetPort=on  CountLoadPort=on  CountEnbPort=on  CountDirPort=off  CountHitOutputPort=off  CountDataType=Unsigned  CountWordLen=16  CountFracLen=0  CountSampTime=1
  Logical Operator : Logic  AllPortsSameDT=off  OutDataTypeStr=boolean
  Logical Operator1 : Logic  AllPortsSameDT=off  OutDataTypeStr=boolean
  Logical Operator2 : Logic  Operator=NOT  AllPortsSameDT=off  OutDataTypeStr=boolean
  Logical Operator3 : Logic  Operator=OR  AllPortsSameDT=off  OutDataTypeStr=boolean
  Logical Operator4 : Logic  Operator=OR  AllPortsSameDT=off  OutDataTypeStr=boolean
  Logical Operator5 : Logic  Operator=OR  AllPortsSameDT=off  OutDataTypeStr=boolean
  Logical Operator6 : Logic  AllPortsSameDT=off  OutDataTypeStr=boolean
  Relational Operator : RelationalOperator  Operator===  OutDataTypeStr=boolean  RndMeth=Simplest  InputSameDT=off
  Relational Operator1 : RelationalOperator  Operator===  OutDataTypeStr=boolean  RndMeth=Simplest  InputSameDT=off
  Simple Dual Port RAM : hdlsllib/HDL RAMs/Simple Dual Port RAM  ram_size=16
  Simple Dual Port RAM1 : hdlsllib/HDL RAMs/Simple Dual Port RAM  ram_size=16
  Switch : Switch  Criteria=u2 > Threshold  SaturateOnIntegerOverflow=off  InputSameDT=off
  dataOut : Outport
  validOut : Outport  Port=2
  wires:
  enb/1 -> HDL Counter/2, Logical Operator6/2, Logical Operator/1, Logical Operator1/1
  Simple Dual Port RAM/1 -> Switch/1
  bps/1 -> 2-D Lookup Table/1
  HDL Counter/1 -> Delay3/1, Relational Operator/1, Delay6/1
  HDL Counter1/1 -> Compare To Constant1/1
  wr_din/1 -> Delay2/1
  Relational Operator/1 -> Logical Operator6/1
  Logical Operator1/1 -> Delay7/1
  2-D Lookup Table/1 -> Delay8/1
  rst/1 -> HDL Counter1/1, Logical Operator4/1, Delay/1
  Simple Dual Port RAM1/1 -> Switch/3
  Logical Operator/1 -> Delay4/1
  Switch/1 -> dataOut/1
  Delay1/1 -> validOut/1
  HDL Counter2/1 -> Compare To Zero/1, Relational Operator1/1, 2-D Lookup Table/2
  Compare To Constant1/1 -> Logical Operator/2, Logical Operator2/1
  numSCs/1 -> Relational Operator1/2, Relational Operator/2
  Relational Operator1/1 -> Logical Operator3/2
  Logical Operator3/1 -> HDL Counter2/1
  Logical Operator4/1 -> HDL Counter/1
  Constant/1 -> HDL Counter2/3
  Compare To Zero/1 -> Logical Operator5/2, HDL Counter2/4
  Logical Operator5/1 -> Delay9/1
  Logical Operator2/1 -> Logical Operator1/2, Delay5/1
  Logical Operator6/1 -> HDL Counter1/2, Logical Operator4/2, Logical Operator5/1, HDL Counter2/2
  Delay/1 -> Logical Operator3/1
  Delay2/1 -> Simple Dual Port RAM1/1, Simple Dual Port RAM/1
  Delay3/1 -> Simple Dual Port RAM/2
  Delay4/1 -> Simple Dual Port RAM/3
  Delay5/1 -> Switch/2
  Delay6/1 -> Simple Dual Port RAM1/2
  Delay7/1 -> Simple Dual Port RAM1/3
  Delay8/1 -> Simple Dual Port RAM/4, Simple Dual Port RAM1/4
  Delay9/1 -> Delay1/1

== system soc_WLAN_fpga/WLAN/WLAN HDL/WLAN_Tx_Rx/WLAN_Rx/WLANHDLReceiver/DataRecovery/Deinterleaver/DeInterleaver_NonHT/ctrlGen ==
  enb : Inport
  numSCs : Inport  Port=2
  rst : Inport  Port=3
  Compare To Zero : simulink/Logic and Bit Operations/Compare To Zero  relop===  OutDataTypeStr=boolean
  HDL Counter : hdlsllib/Sources/HDL Counter  CountType=Count limited  CountInit=0  CountStep=1  CountMax=length(secondPIdx_NonHT)-1  CountFromType=Initial value  CountFrom=0  CountResetPort=on  CountLoadPort=off  CountEnbPort=on  CountDirPort=off  CountHitOutputPort=off  CountDataType=Unsigned  CountWordLen=16  CountFracLen=0  CountSampTime=1
  Logical Operator : Logic  AllPortsSameDT=off  OutDataTypeStr=boolean
  Logical Operator1 : Logic  AllPortsSameDT=off  OutDataTypeStr=boolean
  Logical Operator2 : Logic  Operator=OR  AllPortsSameDT=off  OutDataTypeStr=boolean
  Relational Operator : RelationalOperator  Operator===  OutDataTypeStr=boolean  RndMeth=Simplest  InputSameDT=off
  Out1 : Outport
  Out2 : Outport  Port=2
  wires:
  Logical Operator/1 -> Out2/1
  HDL Counter/1 -> Relational Operator/1, Compare To Zero/1
  Logical Operator1/1 -> Out1/1
  Compare To Zero/1 -> Logical Operator1/2
  enb/1 -> HDL Counter/2, Logical Operator/2, Logical Operator1/1
  Relational Operator/1 -> Logical Operator2/2, Logical Operator/1
  numSCs/1 -> Relational Operator/2
  Logical Operator2/1 -> HDL Counter/1
  rst/1 -> Logical Operator2/1

== system soc_WLAN_fpga/WLAN/WLAN HDL/WLAN_Tx_Rx/WLAN_Rx/WLANHDLReceiver/DataRecovery/Deinterleaver/DeInterleaver_NonHT/numSCsConverter ==
  numSCs : Inport
  bps : Inport  Port=2
  Add : Sum  Inputs=+-
  Add1 : Sum  Inputs=+-
  Add2 : Sum  Inputs=+-
  Add3 : Sum  OutDataTypeStr=fixdt(0,9,0)
  Constant1 : Constant  Value=fi(1,0,1,0)  SampleTime=-1
  Constant3 : Constant  Value=fi(6,0,3,0)  SampleTime=-1
  Multiport Switch5 : MultiPortSwitch  Inputs=4  SaturateOnIntegerOverflow=off  InputSameDT=off
  Product : Product
  Shift Arithmetic : ArithShift  BitShiftNumber=1  BitShiftDirection=Left
  Shift Arithmetic1 : ArithShift  BitShiftNumber=2  BitShiftDirection=Left
  numSCsOut : Outport
  wires:
  Shift Arithmetic/1 -> Add/1
  Multiport Switch5/1 -> numSCsOut/1
  Add2/1 -> Multiport Switch5/5
  Constant1/1 -> Add/2, Add2/2, Add3/2, Add1/2
  bps/1 -> Multiport Switch5/1
  Add1/1 -> Multiport Switch5/4
  Add/1 -> Multiport Switch5/3
  Shift Arithmetic1/1 -> Add1/1
  Constant3/1 -> Product/2
  Product/1 -> Add2/1
  Add3/1 -> Shift Arithmetic/1, Product/1, Shift Arithmetic1/1
  numSCs/1 -> Multiport Switch5/2, Add3/1

== system soc_WLAN_fpga/WLAN/WLAN HDL/WLAN_Tx_Rx/WLAN_Rx/WLANHDLReceiver/FrameFormatDetectionAndSignalRecovery/CRCCheckAndBitInterpretation/numOFDMSymbolCalVHT/rxTimeVHT ==
  note: Calculate the Rx time from L-sig bits for VHT frame format
  In1 : Inport
  Add Constant : Bias  Bias=3  SaturateOnIntegerOverflow=off
  Add Constant1 : Bias  Bias=20  SaturateOnIntegerOverflow=off
  Data Type Conversion : DataTypeConversion  OutDataTypeStr=uint16  RndMeth=Ceiling  SaturateOnIntegerOverflow=off
  Delay : Delay  DelayLength=1
  Delay1 : Delay  DelayLength=1
  Delay2 : Delay  DelayLength=1
  Gain : Gain  Gain=4/3  ParamDataTypeStr=fixdt(1,16,14)
  Out1 : Outport
  wires:
  Add Constant1/1 -> Data Type Conversion/1
  Add Constant/1 -> Delay1/1
  Gain/1 -> Delay2/1
  Data Type Conversion/1 -> Out1/1
  In1/1 -> Delay/1
  Delay/1 -> Add Constant/1
  Delay1/1 -> Gain/1
  Delay2/1 -> Add Constant1/1

== system soc_WLAN_fpga/WLAN/WLAN HDL/WLAN_Tx_Rx/WLAN_Rx/WLANHDLReceiver/FrameFormatDetectionAndSignalRecovery/SignalBitRecovery/Deinterleaver Block/Generate Ready ==
  advPop : Inport
  fifoCount : Inport  Port=2
  pop : Inport  Port=3
  endReady : Inport  Port=4
  Generate Ready2 : Subsystem
  Logical Operator1 : Logic  IconShape=distinctive  AllPortsSameDT=off  OutDataTypeStr=boolean
  Logical Operator2 : Logic  IconShape=distinctive  AllPortsSameDT=off  OutDataTypeStr=boolean
  Logical Operator3 : Logic  Operator=NOT  IconShape=distinctive  AllPortsSameDT=off  OutDataTypeStr=boolean
  MATLAB Function1 : MATLAB Function  TreatAsAtomicUnit=on  mask{nClocks=4}
      mask prompts: nClocks "Number of clocks to hold:"
  ready : Outport
  wires:
  pop/1 -> Generate Ready2/2(pop)
  Logical Operator3/1 -> Logical Operator2/2
  endReady/1 -> Logical Operator1/2
  MATLAB Function1/1(out) -> Logical Operator3/1
  fifoCount/1 -> Generate Ready2/1(fifoCount)
  Logical Operator1/1 -> MATLAB Function1/1(trigger)
  advPop/1 -> Logical Operator1/1
  Logical Operator2/1 -> ready/1
  Generate Ready2/1(ready2) -> Logical Operator2/1

== system soc_WLAN_fpga/WLAN/WLAN HDL/WLAN_Tx_Rx/WLAN_Rx/WLANHDLReceiver/FrameFormatDetectionAndSignalRecovery/SignalBitRecovery/Deinterleaver Block/Read Logic ==
  fifoData : Inport
  fifoCount : Inport  Port=2
  Add1 : Sum  OutDataTypeStr=Inherit: Inherit via back propagation
  Delay1 : Delay  DelayLength=5
  Delay2 : Delay  DelayLength=5
  Delay3 : Delay  DelayLength=1
  Delay4 : Delay  DelayLength=5
  Delay7 : Delay  DelayLength=1
  Generate Base Read Address : Subsystem
  Generate Output Control Signals : Subsystem
  Generate Read Address : Subsystem  Variant=on
  MATLAB Function : MATLAB Function  TreatAsAtomicUnit=on  mask{nClocks=maxBlkSize}
      mask prompts: nClocks "Number of clocks to hold:"
  Relational Operator1 : RelationalOperator  Operator=<  OutDataTypeStr=boolean  InputSameDT=off
  Unit Delay Enabled Synchronous1 : hdlsllib/Discrete/Unit Delay Enabled Synchronous  InitialCondition=maxBlkSize -1  SampleTime=-1
  rdAddr : Outport
  start : Outport  Port=2
  end : Outport  Port=3
  valid : Outport  Port=4
  pop : Outport  Port=5
  advPop : Outport  Port=6
  wires:
  Generate Output Control Signals/5(advPop) -> advPop/1
  Generate Output Control Signals/4(pop) -> pop/1
  Delay1/1 -> Add1/2
  Generate Read Address/1(blockDataCount) -> Generate Output Control Signals/3(blockCount)
  Delay2/1 -> Generate Output Control Signals/2(blockValid)
  Delay4/1 -> Generate Output Control Signals/1(blockLen)
  Delay7/1 -> rdAddr/1
  Generate Output Control Signals/3(valid) -> valid/1
  Generate Output Control Signals/2(end) -> end/1
  Generate Output Control Signals/1(start) -> start/1
  Generate Read Address/2(currentAddr) -> Add1/1
  Generate Base Read Address/1(baseAddr) -> Delay1/1
  fifoData/1 -> Unit Delay Enabled Synchronous1/1
  Add1/1 -> Delay7/1
  Delay3/1 -> Relational Operator1/2
  MATLAB Function/1(out) -> Generate Read Address/2(enable), Delay2/1
  Unit Delay Enabled Synchronous1/1 -> Generate Read Address/1(blockLen), Delay4/1  "blockLen"
  Relational Operator1/1 -> Generate Read Address/3(reset), Generate Base Read Address/1(readStart), Unit Delay Enabled Synchronous1/2, MATLAB Function/1(trigger)  "readStart"
  fifoCount/1 -> Relational Operator1/1, Delay3/1
